simulink model "CLA_Sample"  (R2022b)
settings: Solver=FixedStepAuto  StartTime=0.0  StopTime=Inf  RelTol=1e-3  EnableMultiTasking=on
model workspace (MAT data in the model file):
  ADC_Gain = 1241.21212121
  DAC_Gain = 0.000805860805861
  Inductor_Current_Divider_Gain_Phase_A = 33.4
  Inductor_Current_Divider_Gain_Phase_B = 33.4
  Vbulk_Divider_Gain = 276.854928018
  Vin_Divider_Gain = 556.17352614
undefined symbols (not defined in the file or in its folder): GPTRIP1SEL, GPTRIP2SEL, SCI_A_Transmit, SCI_A_Transmit_Current_Suffix, SCI_A_Transmit_one_shot_Suffix, SCI_A_Transmit_Polarity_Suffix, SCI_A_Transmit_relay_Suffix, SCI_A_Transmit_Vbulk_Suffix, SCI_A_Transmit_Vin_rms_Suffix, SCI_A_Transmit_Vin_Suffix, SCI_A_Transmit_Vmid_Suffix, SCI_A_Transmit_Vp_Suffix, SCI_A_Transmit_Vpfc_Suffix, TZ1, TZ2
libraries: c280xlib x33, simulink x17, c2802xlib x15, c2000lib x1, c2806xlib x1
(part 4 of 5)

== system CLA_Sample/Calibration,RMS, Fault Protection @5kHz/Fault checking/If Action Subsystem/PFC_en_update_Phase_C ==
  function : TriggerPort  TriggerType=function-call  VariantControl=(inherit)
  Chart : Stateflow chart  TreatAsAtomicUnit=on
  Constant : Constant
  Data Store Read : DataStoreRead  Commented=on  DataStoreName=counter_Relay  IndexOptions=Index vector (dialog)  Indices=1  OutputSizes=1
  Data Store Read1 : DataStoreRead  DataStoreName=Vin_UVP_Flag_Phase_C  IndexOptions=Index vector (dialog)  Indices=1  OutputSizes=1
  Data Store Read2 : DataStoreRead  DataStoreName=Vin_OVP_Flag_Phase_C  IndexOptions=Index vector (dialog)  Indices=1  OutputSizes=1
  Data Store Read4 : DataStoreRead  DataStoreName=Iin_OCP_Flag_phase_C  IndexOptions=Index vector (dialog)  Indices=1  OutputSizes=1
  Data Store Write : DataStoreWrite  DataStoreName=PFC_en_Phase_C  IndexOptions=Index vector (dialog)  Indices=1  OutputSizes=1
  Data Store Write1 : DataStoreWrite  DataStoreName=PFC_en1  IndexOptions=Index vector (dialog)  Indices=1  OutputSizes=1
  Data Store Write2 : DataStoreWrite  Commented=on  DataStoreName=counter_Relay  IndexOptions=Index vector (dialog)  Indices=1  OutputSizes=1
  Product : Product  Commented=on
  wires:
  Chart/2(PFC_en1) -> Data Store Write1/1
  Data Store Read1/1 -> Chart/1(Vin_UVP_Flag)
  Data Store Read/1 -> Product/2
  Product/1 -> Data Store Write2/1
  Chart/1(PFC_en) -> Product/1, Data Store Write/1
  Data Store Read2/1 -> Chart/2(Vin_OVP_Flag)
  Data Store Read4/1 -> Chart/3(Iin_OCP_Flag)

== system CLA_Sample/Calibration,RMS, Fault Protection @5kHz/Fault checking/If Action Subsystem/Phase_A_Fault ==
  function : TriggerPort  TriggerType=function-call  VariantControl=(inherit)
  "Fault Check (Input OVP)_Phase_A " : Subsystem  TreatAsAtomicUnit=on
  "Fault Check (Input UVP)_Phase_A " : Subsystem  TreatAsAtomicUnit=on
  Function-Call Generator : simulink/Ports & Subsystems/Function-Call Generator  sample_time=-1  numberOfIterations=1  DisallowWideOutput=off
  Function-Call Split : FunctionCallSplit  IconShape=distinctive  NumOutputPorts=3  OutputPortLayout=default
  Input current_OCP_Phase_A : Subsystem  TreatAsAtomicUnit=on
  wires:
  Function-Call Generator/1 -> Function-Call Split/1
  Function-Call Split/1 -> "Fault Check (Input UVP)_Phase_A "/Trigger
  Function-Call Split/2 -> "Fault Check (Input OVP)_Phase_A "/Trigger
  Function-Call Split/3 -> Input current_OCP_Phase_A/Trigger

== system CLA_Sample/Calibration,RMS, Fault Protection @5kHz/Fault checking/If Action Subsystem/Phase_B_Fault ==
  function : TriggerPort  TriggerType=function-call  VariantControl=(inherit)
  Fault Check (Input OVP)_Phase_B : Subsystem  TreatAsAtomicUnit=on
  Fault Check (Input UVP)_Phase_B : Subsystem  TreatAsAtomicUnit=on
  Function-Call Generator : simulink/Ports & Subsystems/Function-Call Generator  sample_time=-1  numberOfIterations=1  DisallowWideOutput=off
  Function-Call Split : FunctionCallSplit  IconShape=distinctive  NumOutputPorts=3  OutputPortLayout=default
  Input current_OCP_Phase_B : Subsystem  TreatAsAtomicUnit=on
  wires:
  Function-Call Generator/1 -> Function-Call Split/1
  Function-Call Split/1 -> Fault Check (Input UVP)_Phase_B/Trigger
  Function-Call Split/2 -> Fault Check (Input OVP)_Phase_B/Trigger
  Function-Call Split/3 -> Input current_OCP_Phase_B/Trigger

== system CLA_Sample/Calibration,RMS, Fault Protection @5kHz/Fault checking/If Action Subsystem/Phase_C_Fault ==
  function : TriggerPort  TriggerType=function-call  VariantControl=(inherit)
  Fault Check (Input OVP)_Phase_C : Subsystem  TreatAsAtomicUnit=on
  Fault Check (Input UVP)_Phase_C : Subsystem  TreatAsAtomicUnit=on
  Function-Call Generator : simulink/Ports & Subsystems/Function-Call Generator  sample_time=-1  numberOfIterations=1  DisallowWideOutput=off
  Function-Call Split : FunctionCallSplit  IconShape=distinctive  NumOutputPorts=3  OutputPortLayout=default
  Input current_OCP_Phase_C : Subsystem  TreatAsAtomicUnit=on
  wires:
  Function-Call Generator/1 -> Function-Call Split/1
  Function-Call Split/1 -> Fault Check (Input UVP)_Phase_C/Trigger
  Function-Call Split/2 -> Fault Check (Input OVP)_Phase_C/Trigger
  Function-Call Split/3 -> Input current_OCP_Phase_C/Trigger

== system CLA_Sample/Calibration,RMS, Fault Protection @5kHz/Polarity & Near Zero check/Polarity_Near_zero_Phase_A/Volt to Number ==
  In1 : Inport
  Gain : Gain  Gain=ADC_Gain
  Gain1 : Gain  Gain=1/Vin_Divider_Gain
  Out1 : Outport
  wires:
  Gain1/1 -> Gain/1
  In1/1 -> Gain1/1
  Gain/1 -> Out1/1

== system CLA_Sample/Calibration,RMS, Fault Protection @5kHz/Polarity & Near Zero check/Polarity_Near_zero_Phase_B/Volt to Number ==
  In1 : Inport
  Gain : Gain  Gain=ADC_Gain
  Gain1 : Gain  Gain=1/Vin_Divider_Gain
  Out1 : Outport
  wires:
  Gain1/1 -> Gain/1
  In1/1 -> Gain1/1
  Gain/1 -> Out1/1

== system CLA_Sample/Calibration,RMS, Fault Protection @5kHz/Polarity & Near Zero check/Polarity_Near_zero_Phase_C/Volt to Number ==
  In1 : Inport
  Gain : Gain  Gain=ADC_Gain
  Gain1 : Gain  Gain=1/Vin_Divider_Gain
  Out1 : Outport
  wires:
  Gain1/1 -> Gain/1
  In1/1 -> Gain1/1
  Gain/1 -> Out1/1

== system CLA_Sample/Calibration,RMS, Fault Protection @5kHz/Relay control/Subsystem/ADC Gain2 ==
  In1 : Inport
  Gain : Gain  Gain=ADC_Gain
  Gain1 : Gain  Gain=1/Vin_Divider_Gain
  Out1 : Outport
  wires:
  Gain1/1 -> Gain/1
  In1/1 -> Gain1/1
  Gain/1 -> Out1/1

== system CLA_Sample/Calibration,RMS, Fault Protection @5kHz/Relay control/Subsystem/ADC Gain3 ==
  In1 : Inport
  Gain : Gain  Gain=ADC_Gain
  Gain1 : Gain  Gain=1/Vin_Divider_Gain
  Out1 : Outport
  wires:
  Gain1/1 -> Gain/1
  In1/1 -> Gain1/1
  Gain/1 -> Out1/1

== system CLA_Sample/Calibration,RMS, Fault Protection @5kHz/Voltage RMS//Averag Calculation/Phase_A/RMS Current Calculation_Phase_A ==
  note: RMS Voltage Calculation
  function : TriggerPort  TriggerType=function-call  VariantControl=(inherit)
  Chart : Stateflow chart  TreatAsAtomicUnit=on
  Data Store Read2 : DataStoreRead  DataStoreName=Inductor_Current_ADC_Phase_A  IndexOptions=Index vector (dialog)  Indices=1  OutputSizes=1
  Data Store Read5 : DataStoreRead  DataStoreName=Inductor_Current_1_65_ADC_Phase_A  IndexOptions=Index vector (dialog)  Indices=1  OutputSizes=1
  Data Store Write : DataStoreWrite  DataStoreName=Iin_rms_Phase_A  IndexOptions=Index vector (dialog)  Indices=1  OutputSizes=1
  Data Store Write1 : DataStoreWrite  DataStoreName=Iin_peak_Phase_A  IndexOptions=Index vector (dialog)  Indices=1  OutputSizes=1
  Gain1 : Gain  Gain=DAC_Gain
  Gain2 : Gain  Gain=DAC_Gain
  Gain3 : Gain  Gain=Inductor_Current_Divider_Gain_Phase_B
  Gain4 : Gain  Gain=Inductor_Current_Divider_Gain_Phase_B
  Gain5 : Gain  Gain=100
  Gain6 : Gain  Gain=100
  Subtract2 : Sum  Inputs=+-
  wires:
  Data Store Read2/1 -> Subtract2/1
  Data Store Read5/1 -> Subtract2/2
  Subtract2/1 -> Chart/1(input)
  Gain2/1 -> Gain3/1
  Chart/2(Vrms) -> Gain2/1
  Gain3/1 -> Gain6/1
  Gain6/1 -> Data Store Write/1
  Gain4/1 -> Gain5/1
  Gain1/1 -> Gain4/1
  Chart/1(Vpeak) -> Gain1/1
  Gain5/1 -> Data Store Write1/1

== system CLA_Sample/Calibration,RMS, Fault Protection @5kHz/Voltage RMS//Averag Calculation/Phase_A/RMS Voltage Calculation_Phase_A ==
  note: RMS Voltage Calculation
  function : TriggerPort  TriggerType=function-call  VariantControl=(inherit)
  Chart : Stateflow chart  TreatAsAtomicUnit=on
  Data Store Read2 : DataStoreRead  DataStoreName=Vin_ADC_Average_Phase_A  IndexOptions=Index vector (dialog)  Indices=1  OutputSizes=1
  Data Store Read5 : DataStoreRead  DataStoreName=Vin_1_65_ADC_Phase_A  IndexOptions=Index vector (dialog)  Indices=1  OutputSizes=1
  Data Store Write1 : DataStoreWrite  DataStoreName=Vin_peak_Phase_A  IndexOptions=Index vector (dialog)  Indices=1  OutputSizes=1
  Data Store Write2 : DataStoreWrite  DataStoreName=Vin_rms_Phase_A  IndexOptions=Index vector (dialog)  Indices=1  OutputSizes=1
  Data Store Write3 : DataStoreWrite  DataStoreName=Vin_peak_ADC_Phase_A  IndexOptions=Index vector (dialog)  Indices=1  OutputSizes=1
  Data Store Write4 : DataStoreWrite  DataStoreName=Vin_rms_ADC  IndexOptions=Index vector (dialog)  Indices=1  OutputSizes=1
  Digital Output : c280xlib/Digital Output  Commented=on  GPIO_Number=GPIO16~GPIO23  GPIO_Bit0=off  GPIO_BIT0_Toggle=off  GPIO_Bit1=off  GPIO_BIT1_Toggle=off  GPIO_Bit2=off  GPIO_BIT2_Toggle=off  GPIO_Bit3=off  GPIO_BIT3_Toggle=off  GPIO_Bit4=off  GPIO_BIT4_Toggle=off  GPIO_Bit5=off  GPIO_BIT5_Toggle=off  GPIO_Bit6=on  GPIO_BIT6_Toggle=off  GPIO_Bit7=off  GPIO_BIT7_Toggle=off
  Gain6 : Gain  Gain=DAC_Gain
  Gain7 : Gain  Gain=Vin_Divider_Gain  OutDataTypeStr=double
  Gain8 : Gain  Gain=DAC_Gain
  Gain9 : Gain  Gain=Vin_Divider_Gain  OutDataTypeStr=double
  Subtract2 : Sum  Inputs=+-
  wires:
  Chart/1(Vpeak) -> Data Store Write3/1, Gain8/1
  Chart/2(Vrms) -> Gain6/1, Data Store Write4/1
  Gain7/1 -> Data Store Write2/1
  Data Store Read2/1 -> Subtract2/1
  Gain8/1 -> Gain9/1
  Gain6/1 -> Gain7/1
  Data Store Read5/1 -> Subtract2/2
  Gain9/1 -> Data Store Write1/1
  Subtract2/1 -> Chart/1(input)

== system CLA_Sample/Calibration,RMS, Fault Protection @5kHz/Voltage RMS//Averag Calculation/Phase_A/Vin_ADC Averaging_Phase_A ==
  note: Low pass filter :
      | 1kHz bandwidth with 5kHz switching freq
  function : TriggerPort  TriggerType=function-call  VariantControl=(inherit)
  Chart1 : Stateflow chart  TreatAsAtomicUnit=on
  Constant1 : Constant  Value=0.38586954
  Constant2 : Constant  Value=0.38586954
  Constant3 : Constant  Value=-0.22826091
  Data Store Read3 : DataStoreRead  DataStoreName=Vin_ADC_Phase_A  IndexOptions=Index vector (dialog)  Indices=1  OutputSizes=1
  Vin_ADC_Average : DataStoreWrite  DataStoreName=Vin_ADC_Average_Phase_A  IndexOptions=Index vector (dialog)  Indices=1  OutputSizes=1
  wires:
  Constant3/1 -> [a1]
  Constant1/1 -> [b0]
  Constant2/1 -> [b1]
  [a1] -> Chart1/4(a1)
  [b1] -> Chart1/3(b1)
  [b0] -> Chart1/2(b0)
  Data Store Read3/1 -> Chart1/1(input_u)
  Chart1/1(output_y) -> Vin_ADC_Average/1

== system CLA_Sample/Calibration,RMS, Fault Protection @5kHz/Voltage RMS//Averag Calculation/Phase_B/RMS Current Calculation_Phase_B ==
  note: RMS Voltage Calculation
  function : TriggerPort  TriggerType=function-call  VariantControl=(inherit)
  Chart : Stateflow chart  TreatAsAtomicUnit=on
  Data Store Read2 : DataStoreRead  DataStoreName=Inductor_Current_ADC_Phase_B  IndexOptions=Index vector (dialog)  Indices=1  OutputSizes=1
  Data Store Read5 : DataStoreRead  DataStoreName=Inductor_Current_1_65_ADC_Phase_B  IndexOptions=Index vector (dialog)  Indices=1  OutputSizes=1
  Data Store Write : DataStoreWrite  DataStoreName=Iin_rms_Phase_B  IndexOptions=Index vector (dialog)  Indices=1  OutputSizes=1
  Data Store Write1 : DataStoreWrite  DataStoreName=Iin_peak_Phase_B  IndexOptions=Index vector (dialog)  Indices=1  OutputSizes=1
  Gain1 : Gain  Gain=DAC_Gain
  Gain2 : Gain  Gain=DAC_Gain
  Gain3 : Gain  Gain=Inductor_Current_Divider_Gain_Phase_B
  Gain4 : Gain  Gain=Inductor_Current_Divider_Gain_Phase_B
  Gain5 : Gain  Gain=100
  Gain6 : Gain  Gain=100
  Subtract2 : Sum  Inputs=+-
  wires:
  Data Store Read2/1 -> Subtract2/1
  Data Store Read5/1 -> Subtract2/2
  Subtract2/1 -> Chart/1(input)
  Gain2/1 -> Gain3/1
  Chart/2(Vrms) -> Gain2/1
  Gain3/1 -> Gain6/1
  Gain6/1 -> Data Store Write/1
  Gain5/1 -> Data Store Write1/1
  Gain1/1 -> Gain4/1
  Gain4/1 -> Gain5/1
  Chart/1(Vpeak) -> Gain1/1

== system CLA_Sample/Calibration,RMS, Fault Protection @5kHz/Voltage RMS//Averag Calculation/Phase_B/RMS Voltage Calculation_Phase_B ==
  note: RMS Voltage Calculation
  function : TriggerPort  TriggerType=function-call  VariantControl=(inherit)
  Chart : Stateflow chart  TreatAsAtomicUnit=on
  Data Store Read2 : DataStoreRead  DataStoreName=Vin_ADC_Average_Phase_B  IndexOptions=Index vector (dialog)  Indices=1  OutputSizes=1
  Data Store Read5 : DataStoreRead  DataStoreName=Vin_1_65_ADC_Phase_B  IndexOptions=Index vector (dialog)  Indices=1  OutputSizes=1
  Data Store Write1 : DataStoreWrite  DataStoreName=Vin_peak_Phase_B  IndexOptions=Index vector (dialog)  Indices=1  OutputSizes=1
  Data Store Write2 : DataStoreWrite  DataStoreName=Vin_rms_Phase_B  IndexOptions=Index vector (dialog)  Indices=1  OutputSizes=1
  Data Store Write3 : DataStoreWrite  DataStoreName=Vin_peak_ADC_Phase_B  IndexOptions=Index vector (dialog)  Indices=1  OutputSizes=1
  Data Store Write4 : DataStoreWrite  DataStoreName=Vin_rms_ADC  IndexOptions=Index vector (dialog)  Indices=1  OutputSizes=1
  Gain6 : Gain  Gain=DAC_Gain
  Gain7 : Gain  Gain=Vin_Divider_Gain  OutDataTypeStr=double
  Gain8 : Gain  Gain=DAC_Gain
  Gain9 : Gain  Gain=Vin_Divider_Gain  OutDataTypeStr=double
  Subtract2 : Sum  Inputs=+-
  wires:
  Chart/1(Vpeak) -> Data Store Write3/1, Gain8/1
  Chart/2(Vrms) -> Gain6/1, Data Store Write4/1
  Gain7/1 -> Data Store Write2/1
  Data Store Read2/1 -> Subtract2/1
  Gain8/1 -> Gain9/1
  Gain6/1 -> Gain7/1
  Data Store Read5/1 -> Subtract2/2
  Gain9/1 -> Data Store Write1/1
  Subtract2/1 -> Chart/1(input)

== system CLA_Sample/Calibration,RMS, Fault Protection @5kHz/Voltage RMS//Averag Calculation/Phase_B/Vin_ADC Averaging_Phase_B ==
  note: Low pass filter :
      | 1kHz bandwidth with 5kHz switching freq
  function : TriggerPort  TriggerType=function-call  VariantControl=(inherit)
  Chart1 : Stateflow chart  TreatAsAtomicUnit=on
  Constant1 : Constant  Value=0.38586954
  Constant2 : Constant  Value=0.38586954
  Constant3 : Constant  Value=-0.22826091
  Data Store Read3 : DataStoreRead  DataStoreName=Vin_ADC_Phase_B  IndexOptions=Index vector (dialog)  Indices=1  OutputSizes=1
  Vin_ADC_Average : DataStoreWrite  DataStoreName=Vin_ADC_Average_Phase_B  IndexOptions=Index vector (dialog)  Indices=1  OutputSizes=1
  wires:
  Constant3/1 -> [a1]
  Constant1/1 -> [b0]
  Constant2/1 -> [b1]
  [a1] -> Chart1/4(a1)
  [b1] -> Chart1/3(b1)
  [b0] -> Chart1/2(b0)
  Data Store Read3/1 -> Chart1/1(input_u)
  Chart1/1(output_y) -> Vin_ADC_Average/1

== system CLA_Sample/Calibration,RMS, Fault Protection @5kHz/Voltage RMS//Averag Calculation/Phase_C/RMS Current Calculation_Phase_C ==
  note: RMS Voltage Calculation
  function : TriggerPort  TriggerType=function-call  VariantControl=(inherit)
  Chart : Stateflow chart  TreatAsAtomicUnit=on
  Data Store Read2 : DataStoreRead  DataStoreName=Inductor_Current_ADC_Phase_C  IndexOptions=Index vector (dialog)  Indices=1  OutputSizes=1
  Data Store Read5 : DataStoreRead  DataStoreName=Inductor_Current_1_65_ADC_Phase_C  IndexOptions=Index vector (dialog)  Indices=1  OutputSizes=1
  Data Store Write : DataStoreWrite  DataStoreName=Iin_rms_Phase_C  IndexOptions=Index vector (dialog)  Indices=1  OutputSizes=1
  Data Store Write1 : DataStoreWrite  DataStoreName=Iin_peak_Phase_C  IndexOptions=Index vector (dialog)  Indices=1  OutputSizes=1
  Gain1 : Gain  Gain=DAC_Gain
  Gain2 : Gain  Gain=DAC_Gain
  Gain3 : Gain  Gain=Inductor_Current_Divider_Gain_Phase_B
  Gain4 : Gain  Gain=Inductor_Current_Divider_Gain_Phase_B
  Gain5 : Gain  Gain=100
  Gain6 : Gain  Gain=100
  Subtract2 : Sum  Inputs=+-
  wires:
  Data Store Read2/1 -> Subtract2/1
  Data Store Read5/1 -> Subtract2/2
  Subtract2/1 -> Chart/1(input)
  Gain2/1 -> Gain3/1
  Chart/2(Vrms) -> Gain2/1
  Gain3/1 -> Gain6/1
  Gain6/1 -> Data Store Write/1
  Gain5/1 -> Data Store Write1/1
  Gain1/1 -> Gain4/1
  Gain4/1 -> Gain5/1
  Chart/1(Vpeak) -> Gain1/1

== system CLA_Sample/Calibration,RMS, Fault Protection @5kHz/Voltage RMS//Averag Calculation/Phase_C/RMS Voltage Calculation_Phase_C ==
  note: RMS Voltage Calculation
  function : TriggerPort  TriggerType=function-call  VariantControl=(inherit)
  Chart : Stateflow chart  TreatAsAtomicUnit=on
  Data Store Read2 : DataStoreRead  DataStoreName=Vin_ADC_Average_Phase_C  IndexOptions=Index vector (dialog)  Indices=1  OutputSizes=1
  Data Store Read5 : DataStoreRead  DataStoreName=Vin_1_65_ADC_Phase_C  IndexOptions=Index vector (dialog)  Indices=1  OutputSizes=1
  Data Store Write1 : DataStoreWrite  DataStoreName=Vin_peak_Phase_C  IndexOptions=Index vector (dialog)  Indices=1  OutputSizes=1
  Data Store Write2 : DataStoreWrite  DataStoreName=Vin_rms_Phase_C  IndexOptions=Index vector (dialog)  Indices=1  OutputSizes=1
  Data Store Write3 : DataStoreWrite  DataStoreName=Vin_peak_ADC_Phase_C  IndexOptions=Index vector (dialog)  Indices=1  OutputSizes=1
  Data Store Write4 : DataStoreWrite  DataStoreName=Vin_rms_ADC  IndexOptions=Index vector (dialog)  Indices=1  OutputSizes=1
  Gain6 : Gain  Gain=DAC_Gain
  Gain7 : Gain  Gain=Vin_Divider_Gain  OutDataTypeStr=double
  Gain8 : Gain  Gain=DAC_Gain
  Gain9 : Gain  Gain=Vin_Divider_Gain  OutDataTypeStr=double
  Subtract2 : Sum  Inputs=+-
  wires:
  Chart/1(Vpeak) -> Data Store Write3/1, Gain8/1
  Chart/2(Vrms) -> Gain6/1, Data Store Write4/1
  Gain7/1 -> Data Store Write2/1
  Data Store Read2/1 -> Subtract2/1
  Gain8/1 -> Gain9/1
  Gain6/1 -> Gain7/1
  Data Store Read5/1 -> Subtract2/2
  Gain9/1 -> Data Store Write1/1
  Subtract2/1 -> Chart/1(input)

== system CLA_Sample/Calibration,RMS, Fault Protection @5kHz/Voltage RMS//Averag Calculation/Phase_C/Vin_ADC Averaging_Phase_C ==
  note: Low pass filter :
      | 1kHz bandwidth with 5kHz switching freq
  function : TriggerPort  TriggerType=function-call  VariantControl=(inherit)
  Chart1 : Stateflow chart  TreatAsAtomicUnit=on
  Constant1 : Constant  Value=0.38586954
  Constant2 : Constant  Value=0.38586954
  Constant3 : Constant  Value=-0.22826091
  Data Store Read3 : DataStoreRead  DataStoreName=Vin_ADC_Phase_C  IndexOptions=Index vector (dialog)  Indices=1  OutputSizes=1
  Vin_ADC_Average : DataStoreWrite  DataStoreName=Vin_ADC_Average_Phase_C  IndexOptions=Index vector (dialog)  Indices=1  OutputSizes=1
  wires:
  Constant3/1 -> [a1]
  Constant1/1 -> [b0]
  Constant2/1 -> [b1]
  [a1] -> Chart1/4(a1)
  [b1] -> Chart1/3(b1)
  [b0] -> Chart1/2(b0)
  Data Store Read3/1 -> Chart1/1(input_u)
  Chart1/1(output_y) -> Vin_ADC_Average/1

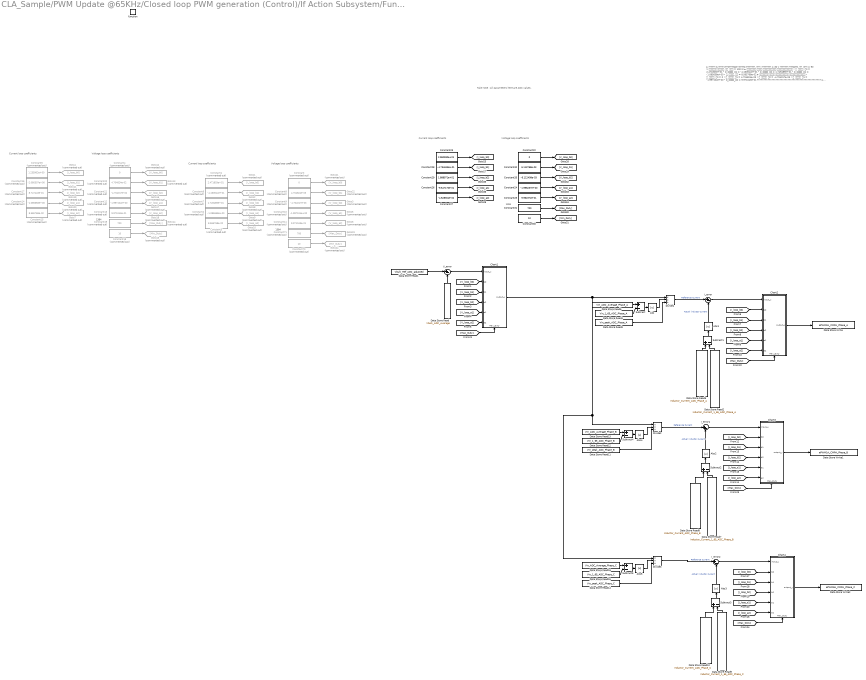
== system CLA_Sample/PWM Update @65KHz/Closed loop PWM generation (Control)/If Action Subsystem/Function-Call Subsystem ==
  note: 1384
  note: Voltage loop coefficients
  note: 1384
  note: Current loop coefficients
  note: Voltage loop coefficients
  note: Voltage loop coefficients
  note: ► 𝑷𝒍𝒂𝒏𝒕 & 𝑳𝒐𝒂𝒅 𝒑𝒂𝒓𝒂𝒎𝒆𝒕𝒆𝒓𝒔
      | 𝑰𝒏𝒑𝒖𝒕 𝒗𝒐𝒍𝒕𝒂𝒈𝒆, 𝑽𝒊𝒏_𝒏𝒐𝒎𝒊𝒏𝒂𝒍 = 30 V
      | 𝑶𝒖𝒕𝒑𝒖𝒕 𝒗𝒐𝒍𝒕𝒂𝒈𝒆, 𝑽𝒐_𝑷𝑭𝑪 = 90 V
      | 𝑶𝒖𝒕𝒑𝒖𝒕 𝒑𝒐𝒘𝒆𝒓, 𝑷𝒐_𝑷𝑭𝑪 = 100 W
      |
      | ► 𝑪𝒖𝒓𝒓𝒆𝒏𝒕 𝒍𝒐𝒐𝒑 𝒄𝒐𝒏𝒕𝒓𝒐𝒍𝒍𝒆𝒓 𝒄𝒐𝒆𝒇𝒇𝒊𝒄𝒊𝒆𝒏𝒕𝒔
      | • 𝑰_𝒍𝒐𝒐𝒑_𝒃0 = 2.471803e+01
      | • 𝑰_𝒍𝒐𝒐𝒑_𝒃1 = -4.160614e+01
      | • 𝑰_𝒍𝒐𝒐𝒑_𝒃2 = 1.749489e+01
      | • 𝑰_𝒍𝒐𝒐𝒑_𝒂1 = -1.085658e+00
      | • 𝑰_𝒍𝒐𝒐𝒑_𝒂2 = 8.565768e-02
      |
      | ► 𝑽𝒐𝒍𝒕𝒂𝒈𝒆 𝒍𝒐𝒐𝒑 𝒄𝒐𝒏𝒕𝒓𝒐𝒍𝒍𝒆𝒓 𝒄𝒐𝒆𝒇𝒇𝒊𝒄𝒊𝒆𝒏𝒕𝒔
      | • 𝑽_𝒍𝒐𝒐𝒑_𝒃0 = 0
      | • 𝑽_𝒍𝒐𝒐𝒑_𝒃1 = 4.704824e-03
      | • 𝑽_𝒍𝒐𝒐𝒑_𝒃2 = -4.704017e-03
      | • 𝑽_𝒍𝒐𝒐𝒑_𝒂1 = -1.997104e+00
      | • 𝑽_𝒍𝒐𝒐𝒑_𝒂2 = 9.971043e-01
      |
      | ************************************************
      | ► 𝑻𝒉𝒆 𝒇𝒐𝒓𝒎𝒂𝒕 𝒇𝒐𝒓 𝒄𝒐𝒆𝒇𝒇𝒊𝒄𝒊𝒆𝒏𝒕𝒔 𝒊𝒔 𝒔𝒉𝒐𝒘𝒏 𝒃𝒆𝒍𝒐𝒘.
      |
      | 𝒚(𝒌) = 𝒃0 𝒆(𝒌) + 𝒃1 𝒆(𝒌−1) + 𝒃2 𝒆(𝒌−2) − 𝒂1 𝒚(𝒌−1) − 𝒂2 𝒚(𝒌−2)
      |
      | ************************************************
      | ◘◘◘◘◘◘◘◘◘◘◘◘◘◘◘◘◘◘◘◘◘◘◘◘◘◘◘◘◘◘◘◘◘◘◘◘◘◘◘◘◘◘◘◘◘◘◘◘
  note: 1384
  note: Current loop coefficients
  note: Take note : All parameters here are ADC values.
  note: Current loop coefficients
  function : TriggerPort  TriggerType=function-call  VariantControl=(inherit)
  Abs{,1..5} (6 alike) : Abs  SaturateOnIntegerOverflow=off
  Chart1 : Stateflow chart  TreatAsAtomicUnit=on
      settings: PortSchema="{\"entries\":[{\"content\":{\"sides\":[{\"content\":{\"connectorIds\":[\"In2\",\"In3\",\"In4\",\"In5\",\"In6\",\"In7\"]},\"type\":\"ConnectorPlacement.EquallySpacedRectSide\",\"uuid\":\"98054acb-dc05-45b7-9e49-d1f1309a60af\"},{\"content\":{\"connectorIds\":[\"Out1\"],\"side\":\"RIGHT\"},\"type\":\"ConnectorPlacement.EquallySpacedRectSide\",\"uuid\":\"519c6a11-fba4-4420-9bc2-f24cec898983\"},{\"content\":{\"connectorIds\":[],\"side\":\"TOP\"},\"type\":\"ConnectorPlacement.EquallySpacedRectSide\",\"uuid\":\"37e92206-8070-4c6c-85b3-8eb12c5538cd\"},{\"content\":{\"connectorIds\":[\"In1\"],\"side\":\"BOTTOM\"},\"type\":\"ConnectorPlacement.EquallySpacedRectSide\",\"uuid\":\"a24e42b6-e88f-4c7d-a70a-f75d0d02a985\"}]},\"type\":\"ConnectorPlacement.EquallySpacedConnector\",\"uuid\":\"7d467722-ac20-43d4-98e5-7341f60d2894\"}],\"packageUris\":[\"http://schema.mathworks.com/mf0/Connector/R2020b\"],\"version\":\"1.0\"}"
  Chart2 : Stateflow chart  TreatAsAtomicUnit=on
      settings: PortSchema="{\"entries\":[{\"content\":{\"sides\":[{\"content\":{\"connectorIds\":[\"In2\",\"In3\",\"In4\",\"In5\",\"In6\",\"In7\"]},\"type\":\"ConnectorPlacement.EquallySpacedRectSide\",\"uuid\":\"98054acb-dc05-45b7-9e49-d1f1309a60af\"},{\"content\":{\"connectorIds\":[\"Out1\"],\"side\":\"RIGHT\"},\"type\":\"ConnectorPlacement.EquallySpacedRectSide\",\"uuid\":\"519c6a11-fba4-4420-9bc2-f24cec898983\"},{\"content\":{\"connectorIds\":[],\"side\":\"TOP\"},\"type\":\"ConnectorPlacement.EquallySpacedRectSide\",\"uuid\":\"37e92206-8070-4c6c-85b3-8eb12c5538cd\"},{\"content\":{\"connectorIds\":[\"In1\"],\"side\":\"BOTTOM\"},\"type\":\"ConnectorPlacement.EquallySpacedRectSide\",\"uuid\":\"c357f4bc-ad64-4f69-8a5c-2d122a217843\"}]},\"type\":\"ConnectorPlacement.EquallySpacedConnector\",\"uuid\":\"7d467722-ac20-43d4-98e5-7341f60d2894\"}],\"packageUris\":[\"http://schema.mathworks.com/mf0/Connector/R2020b\"],\"version\":\"1.0\"}"
  Chart3 : Stateflow chart  TreatAsAtomicUnit=on
      settings: PortSchema="{\"entries\":[{\"content\":{\"sides\":[{\"content\":{\"connectorIds\":[\"In2\",\"In3\",\"In4\",\"In5\",\"In6\",\"In7\"]},\"type\":\"ConnectorPlacement.EquallySpacedRectSide\",\"uuid\":\"98054acb-dc05-45b7-9e49-d1f1309a60af\"},{\"content\":{\"connectorIds\":[\"Out1\"],\"side\":\"RIGHT\"},\"type\":\"ConnectorPlacement.EquallySpacedRectSide\",\"uuid\":\"519c6a11-fba4-4420-9bc2-f24cec898983\"},{\"content\":{\"connectorIds\":[],\"side\":\"TOP\"},\"type\":\"ConnectorPlacement.EquallySpacedRectSide\",\"uuid\":\"37e92206-8070-4c6c-85b3-8eb12c5538cd\"},{\"content\":{\"connectorIds\":[\"In1\"],\"side\":\"BOTTOM\"},\"type\":\"ConnectorPlacement.EquallySpacedRectSide\",\"uuid\":\"2f414d73-99cb-441b-a85c-e16df8718e53\"}]},\"type\":\"ConnectorPlacement.EquallySpacedConnector\",\"uuid\":\"7d467722-ac20-43d4-98e5-7341f60d2894\"}],\"packageUris\":[\"http://schema.mathworks.com/mf0/Connector/R2020b\"],\"version\":\"1.0\"}"
  Chart4 : Stateflow chart  TreatAsAtomicUnit=on
      settings: PortSchema="{\"entries\":[{\"content\":{\"sides\":[{\"content\":{\"connectorIds\":[\"In2\",\"In3\",\"In4\",\"In5\",\"In6\",\"In7\"]},\"type\":\"ConnectorPlacement.EquallySpacedRectSide\",\"uuid\":\"98054acb-dc05-45b7-9e49-d1f1309a60af\"},{\"content\":{\"connectorIds\":[\"Out1\"],\"side\":\"RIGHT\"},\"type\":\"ConnectorPlacement.EquallySpacedRectSide\",\"uuid\":\"519c6a11-fba4-4420-9bc2-f24cec898983\"},{\"content\":{\"connectorIds\":[],\"side\":\"TOP\"},\"type\":\"ConnectorPlacement.EquallySpacedRectSide\",\"uuid\":\"37e92206-8070-4c6c-85b3-8eb12c5538cd\"},{\"content\":{\"connectorIds\":[\"In1\"],\"side\":\"BOTTOM\"},\"type\":\"ConnectorPlacement.EquallySpacedRectSide\",\"uuid\":\"3fbeedd5-4cc1-4149-822b-0a6b54a0fe71\"}]},\"type\":\"ConnectorPlacement.EquallySpacedConnector\",\"uuid\":\"7d467722-ac20-43d4-98e5-7341f60d2894\"}],\"packageUris\":[\"http://schema.mathworks.com/mf0/Connector/R2020b\"],\"version\":\"1.0\"}"
  Constant : Constant  Commented=on  Value=0
  Constant1 : Constant  Commented=on  Value=2.471803e+01
  Constant10 : Constant  Commented=on  Value=-1.997104e+00
  Constant11 : Constant  Commented=on  Value=9.971043e-01
  Constant12 : Constant  Commented=on  Value=-1.997104e+00
  Constant13 : Constant  Commented=on  Value=9.971043e-01
  Constant14 : Constant  Commented=on  Value=-1.085658e+00
  Constant15 : Constant  Commented=on  Value=8.565768e-02
  Constant16 : Constant  Commented=on  Value=-2.080307e+00
  Constant17 : Constant  Commented=on  Value=8.747443e-01
  Constant18 : Constant  Commented=on  Value=10  OutDataTypeStr=double
  Constant19 : Constant  Commented=on  Value=700  OutDataTypeStr=double
  Constant2 : Constant  Commented=on  Value=-1.085658e+00
  Constant20 : Constant  Commented=on  Value=4.704824e-02
  Constant21 : Constant  Commented=on  Value=-4.704017e-02
  Constant22 : Constant  Value=0
  Constant23 : Constant  Value=2.962930e+01
  Constant24 : Constant  Value=-1.996237e+00
  Constant25 : Constant  Value=9.962372e-01
  Constant26 : Constant  Value=-9.547170e-01
  Constant27 : Constant  Value=-4.528304e-02
  Constant28 : Constant  Value=-4.734618e+01
  Constant29 : Constant  Value=1.888971e+01
  Constant3 : Constant  Commented=on  Value=8.565768e-02
  Constant30 : Constant  Value=10  OutDataTypeStr=double
  Constant31 : Constant  Value=700  OutDataTypeStr=double
  Constant32 : Constant  Value=6.113768e-03
  Constant33 : Constant  Value=-6.112408e-03
  Constant4 : Constant  Commented=on  Value=0
  Constant5 : Constant  Commented=on  Value=1.235902e+00
  Constant6 : Constant  Commented=on  Value=-4.160614e+01
  Constant7 : Constant  Commented=on  Value=1.749489e+01
  Constant70 : Constant  Commented=on  Value=10  OutDataTypeStr=double
  Constant71 : Constant  Commented=on  Value=700  OutDataTypeStr=double
  Constant8 : Constant  Commented=on  Value=4.704824e-03
  Constant9 : Constant  Commented=on  Value=-4.704017e-03
  Data Store Read : DataStoreRead  DataStoreName=Vbulk_ADC_Average  IndexOptions=Index vector (dialog)  Indices=1  OutputSizes=1
  Data Store Read1 : DataStoreRead  DataStoreName=Vbulk_Ref_ADC_adjusted  IndexOptions=Index vector (dialog)  Indices=1  OutputSizes=1
  Data Store Read10 : DataStoreRead  DataStoreName=Inductor_Current_ADC_Phase_C  IndexOptions=Index vector (dialog)  Indices=1  OutputSizes=1
  Data Store Read11 : DataStoreRead  DataStoreName=Vin_peak_ADC_Phase_B  IndexOptions=Index vector (dialog)  Indices=1  OutputSizes=1
  Data Store Read12 : DataStoreRead  DataStoreName=Vin_1_65_ADC_Phase_B  IndexOptions=Index vector (dialog)  Indices=1  OutputSizes=1
  Data Store Read13 : DataStoreRead  DataStoreName=Vin_ADC_Average_Phase_B  IndexOptions=Index vector (dialog)  Indices=1  OutputSizes=1
  Data Store Read14 : DataStoreRead  DataStoreName=Vin_peak_ADC_Phase_C  IndexOptions=Index vector (dialog)  Indices=1  OutputSizes=1
  Data Store Read15 : DataStoreRead  DataStoreName=Vin_1_65_ADC_Phase_C  IndexOptions=Index vector (dialog)  Indices=1  OutputSizes=1
  Data Store Read16 : DataStoreRead  DataStoreName=Vin_ADC_Average_Phase_C  IndexOptions=Index vector (dialog)  Indices=1  OutputSizes=1
  Data Store Read2 : DataStoreRead  DataStoreName=Inductor_Current_1_65_ADC_Phase_A  IndexOptions=Index vector (dialog)  Indices=1  OutputSizes=1
  Data Store Read3 : DataStoreRead  DataStoreName=Vin_peak_ADC_Phase_A  IndexOptions=Index vector (dialog)  Indices=1  OutputSizes=1
  Data Store Read4 : DataStoreRead  DataStoreName=Vin_1_65_ADC_Phase_A  IndexOptions=Index vector (dialog)  Indices=1  OutputSizes=1
  Data Store Read5 : DataStoreRead  DataStoreName=Inductor_Current_ADC_Phase_A  IndexOptions=Index vector (dialog)  Indices=1  OutputSizes=1
  Data Store Read6 : DataStoreRead  DataStoreName=Vin_ADC_Average_Phase_A  IndexOptions=Index vector (dialog)  Indices=1  OutputSizes=1
  Data Store Read7 : DataStoreRead  DataStoreName=Inductor_Current_1_65_ADC_Phase_B  IndexOptions=Index vector (dialog)  Indices=1  OutputSizes=1
  Data Store Read8 : DataStoreRead  DataStoreName=Inductor_Current_ADC_Phase_B  IndexOptions=Index vector (dialog)  Indices=1  OutputSizes=1
  Data Store Read9 : DataStoreRead  DataStoreName=Inductor_Current_1_65_ADC_Phase_C  IndexOptions=Index vector (dialog)  Indices=1  OutputSizes=1
  Data Store Write : DataStoreWrite  DataStoreName=ePWM2A_CMPA_Phase_A  IndexOptions=Index vector (dialog)  Indices=1  OutputSizes=1
  Data Store Write1 : DataStoreWrite  DataStoreName=ePWM1A_CMPA_Phase_B  IndexOptions=Index vector (dialog)  Indices=1  OutputSizes=1
  Data Store Write2 : DataStoreWrite  DataStoreName=ePWM3A_CMPA_Phase_C  IndexOptions=Index vector (dialog)  Indices=1  OutputSizes=1
  Divide1 : Product  Inputs=**/  RndMeth=Zero  SaturateOnIntegerOverflow=on
  Divide2 : Product  Inputs=**/  RndMeth=Zero  SaturateOnIntegerOverflow=on
  Divide3 : Product  Inputs=**/  RndMeth=Zero  SaturateOnIntegerOverflow=on
  Goto1 : Goto  Commented=on  GotoTag=I_loop_b0
  Goto10 : Goto  Commented=on  GotoTag=I_loop_a2
  Goto11 : Goto  Commented=on  GotoTag=I_loop_b1
  Goto12 : Goto  Commented=on  GotoTag=V_loop_b0
  Goto13 : Goto  Commented=on  GotoTag=V_loop_b1
  Goto14 : Goto  Commented=on  GotoTag=Max_Duty
  Goto15 : Goto  Commented=on  GotoTag=Min_Duty
  Goto16 : Goto  Commented=on  GotoTag=V_loop_b2
  Goto17 : Goto  Commented=on  GotoTag=V_loop_a1
  Goto18 : Goto  Commented=on  GotoTag=V_loop_a2
  Goto19 : Goto  Commented=on  GotoTag=I_loop_b2
  Goto2 : Goto  Commented=on  GotoTag=I_loop_b1
  Goto20 : Goto  Commented=on  GotoTag=I_loop_a1
  Goto21 : Goto  Commented=on  GotoTag=V_loop_b0
  Goto22 : Goto  Commented=on  GotoTag=V_loop_b1
  Goto23 : Goto  Commented=on  GotoTag=Max_Duty
  Goto24 : Goto  Commented=on  GotoTag=Min_Duty
  Goto3 : Goto  Commented=on  GotoTag=V_loop_b2
  Goto4 : Goto  Commented=on  GotoTag=I_loop_b0
  Goto5 : Goto  Commented=on  GotoTag=V_loop_a1
  Goto6 : Goto  Commented=on  GotoTag=V_loop_a2
  Goto7 : Goto  Commented=on  GotoTag=I_loop_a2
  Goto8 : Goto  Commented=on  GotoTag=I_loop_b2
  Goto9 : Goto  Commented=on  GotoTag=I_loop_a1
  I_error : Sum  Inputs=|+-  AccumDataTypeStr=double  OutDataTypeStr=double
  I_error1 : Sum  Inputs=|+-  AccumDataTypeStr=double  OutDataTypeStr=double
  I_error2 : Sum  Inputs=|+-  AccumDataTypeStr=double  OutDataTypeStr=double
  Subtract{,1..5} (6 alike) : Sum  Inputs=+-
  V_error : Sum  Inputs=|+-  AccumDataTypeStr=double  OutDataTypeStr=double
  wires:
  Divide1/1 -> I_error/1  "Reference Current"
  [I_loop_a1] -> Chart4/6(a1)
  Chart1/1(output_y) -> Divide3/1, Divide2/1, Divide1/1
  Data Store Read5/1 -> Subtract1/1
  Constant22/1 -> [V_loop_b0]
  Constant32/1 -> [V_loop_b1]
  I_error2/1 -> Chart4/2(input_u)
  Subtract4/1 -> Abs4/1
  Constant14/1 -> Goto20/1
  Data Store Read11/1 -> Divide2/3
  Subtract5/1 -> Abs5/1
  Abs2/1 -> I_error1/2  "Actual inductor current"
  Constant25/1 -> [V_loop_a2]
  Data Store Read14/1 -> Divide3/3
  Data Store Read15/1 -> Subtract5/2
  Abs5/1 -> Divide3/2
  Divide3/1 -> I_error2/1  "Reference Current"
  [I_loop_b0] -> Chart3/3(b0)
  Constant33/1 -> [V_loop_b2]
  Constant71/1 -> Goto23/1
  [I_loop_b0] -> Chart2/3(b0)
  [V_loop_a1] -> Chart1/6(a1)
  Constant6/1 -> Goto2/1
  Subtract1/1 -> Abs1/1
  [V_loop_b2] -> Chart1/5(b2)
  Abs4/1 -> Divide2/2
  Constant/1 -> Goto21/1
  Chart4/1(output_y) -> Data Store Write2/1
  Data Store Read7/1 -> Subtract2/2
  Data Store Read8/1 -> Subtract2/1
  [I_loop_a2] -> Chart3/7(a2)
  Chart2/1(output_y) -> Data Store Write/1
  [I_loop_b2] -> Chart3/5(b2)
  [I_loop_b1] -> Chart3/4(b1)
  Data Store Read1/1 -> V_error/1
  [I_loop_a2] -> Chart2/7(a2)
  Subtract2/1 -> Abs2/1
  Constant10/1 -> Goto5/1
  Abs1/1 -> I_error/2  "Actual inductor current"
  Data Store Read2/1 -> Subtract1/2
  Subtract/1 -> Abs/1
  Constant2/1 -> Goto9/1
  Constant3/1 -> Goto10/1
  Constant9/1 -> Goto3/1
  Constant11/1 -> Goto6/1
  Constant8/1 -> Goto22/1
  Data Store Read4/1 -> Subtract/2
  Constant7/1 -> Goto8/1
  [I_loop_b1] -> Chart2/4(b1)
  Chart3/1(output_y) -> Data Store Write1/1
  [V_loop_b0] -> Chart1/3(b0)
  [Max_Duty] -> Chart3/1(Max_Duty)
  Data Store Read3/1 -> Divide1/3
  Constant70/1 -> Goto24/1
  Constant20/1 -> Goto13/1
  Data Store Read9/1 -> Subtract3/2
  Data Store Read10/1 -> Subtract3/1
  [I_loop_b0] -> Chart4/3(b0)
  [V_loop_a2] -> Chart1/7(a2)
  Constant13/1 -> Goto18/1
  [V_loop_b1] -> Chart1/4(b1)
  V_error/1 -> Chart1/2(input_u)
  [I_loop_a2] -> Chart4/7(a2)
  Constant16/1 -> Goto11/1
  [I_loop_a1] -> Chart2/6(a1)
  Constant21/1 -> Goto16/1
  [I_loop_a1] -> Chart3/6(a1)
  Constant15/1 -> Goto7/1
  Abs3/1 -> I_error2/2  "Actual inductor current"
  Constant12/1 -> Goto17/1
  Divide2/1 -> I_error1/1  "Reference Current"
  I_error/1 -> Chart2/2(input_u)
  Constant27/1 -> [I_loop_a2]
  Constant31/1 -> [Max_Duty]
  Subtract3/1 -> Abs3/1
  [Max_Duty] -> Chart1/1(Max_Duty)
  Constant5/1 -> Goto4/1
  I_error1/1 -> Chart3/2(input_u)
  [I_loop_b1] -> Chart4/4(b1)
  Constant18/1 -> Goto15/1
  [Max_Duty] -> Chart4/1(Max_Duty)
  Constant28/1 -> [I_loop_b1]
  [I_loop_b2] -> Chart2/5(b2)
  [Max_Duty] -> Chart2/1(Max_Duty)
  Constant26/1 -> [I_loop_a1]
  Data Store Read6/1 -> Subtract/1
  Constant30/1 -> [Min_Duty]
  Constant29/1 -> [I_loop_b2]
  Data Store Read13/1 -> Subtract4/1
  Constant19/1 -> Goto14/1
  Data Store Read/1 -> V_error/2
  Abs/1 -> Divide1/2
  Constant24/1 -> [V_loop_a1]
  Constant23/1 -> [I_loop_b0]
  Data Store Read16/1 -> Subtract5/1
  [I_loop_b2] -> Chart4/5(b2)
  Constant1/1 -> Goto1/1
  Data Store Read12/1 -> Subtract4/2
  Constant4/1 -> Goto12/1
  Constant17/1 -> Goto19/1

== system CLA_Sample/PWM Update @65KHz/Fixed Duty update_Phase_A/Archive/If Action Subsystem ==
  Action Port : ActionPort  ActionPortLabel=if(u1 ==0)
  Constant : Constant  Value=0
  Data Store Write : DataStoreWrite  DataStoreName=PWM_DutyNearzero  IndexOptions=Index vector (dialog)  Indices=1  OutputSizes=1
  wires:
  Constant/1 -> Data Store Write/1

== system CLA_Sample/PWM Update @65KHz/Fixed Duty update_Phase_A/Archive/If Action Subsystem1 ==
  In1 : Inport  OutDataTypeStr=double
  Action Port : ActionPort  ActionPortLabel=if(u1 ==1)
  Out1 : Outport  OutDataTypeStr=double
  wires:
  In1/1 -> Out1/1

== system CLA_Sample/PWM Update @65KHz/Fixed Duty update_Phase_A/Archive/If Action Subsystem2 ==
  In1 : Inport
  Action Port : ActionPort  ActionPortLabel=else
  Out1 : Outport
  wires:
  In1/1 -> Out1/1

== system CLA_Sample/PWM Update @65KHz/Fixed Duty update_Phase_A/Archive/If Action Subsystem3 ==
  Action Port : ActionPort  ActionPortLabel=else
  Data Store Read7 : DataStoreRead  DataStoreName=Polarity_Phase_A  IndexOptions=Index vector (dialog)  Indices=1  OutputSizes=1
  If Action Subsystem4 : Subsystem  TreatAsAtomicUnit=on
  If Action Subsystem5 : Subsystem  TreatAsAtomicUnit=on
  If2 : If  IfExpression=u1 ==1
  wires:
  Data Store Read7/1 -> If2/1
  If2/2 -> If Action Subsystem5/Action
  If2/1 -> If Action Subsystem4/Action

== system CLA_Sample/PWM Update @65KHz/Fixed Duty update_Phase_B/Archive/If Action Subsystem ==
  Action Port : ActionPort
  Constant : Constant  Value=0
  Data Store Write : DataStoreWrite  DataStoreName=PWM_DutyNearzero  IndexOptions=Index vector (dialog)  Indices=1  OutputSizes=1
  wires:
  Constant/1 -> Data Store Write/1

== system CLA_Sample/PWM Update @65KHz/Fixed Duty update_Phase_B/Archive/If Action Subsystem1 ==
  In1 : Inport  OutDataTypeStr=double
  Action Port : ActionPort
  Out1 : Outport  OutDataTypeStr=double
  wires:
  In1/1 -> Out1/1

== system CLA_Sample/PWM Update @65KHz/Fixed Duty update_Phase_B/Archive/If Action Subsystem2 ==
  In1 : Inport
  Action Port : ActionPort
  Out1 : Outport
  wires:
  In1/1 -> Out1/1

== system CLA_Sample/PWM Update @65KHz/Fixed Duty update_Phase_B/Archive/If Action Subsystem3 ==
  Action Port : ActionPort
  Data Store Read7 : DataStoreRead  DataStoreName=Polarity_Phase_A  IndexOptions=Index vector (dialog)  Indices=1  OutputSizes=1
  If Action Subsystem4 : Subsystem  TreatAsAtomicUnit=on
  If Action Subsystem5 : Subsystem  TreatAsAtomicUnit=on
  If2 : If  IfExpression=u1 ==1
  wires:
  Data Store Read7/1 -> If2/1
  If2/2 -> If Action Subsystem5/Action
  If2/1 -> If Action Subsystem4/Action

== system CLA_Sample/PWM Update @65KHz/Fixed Duty update_Phase_C/Archive/If Action Subsystem ==
  Action Port : ActionPort
  Constant : Constant  Value=0
  Data Store Write : DataStoreWrite  DataStoreName=PWM_DutyNearzero  IndexOptions=Index vector (dialog)  Indices=1  OutputSizes=1
  wires:
  Constant/1 -> Data Store Write/1

== system CLA_Sample/PWM Update @65KHz/Fixed Duty update_Phase_C/Archive/If Action Subsystem1 ==
  In1 : Inport  OutDataTypeStr=double
  Action Port : ActionPort
  Out1 : Outport  OutDataTypeStr=double
  wires:
  In1/1 -> Out1/1

== system CLA_Sample/PWM Update @65KHz/Fixed Duty update_Phase_C/Archive/If Action Subsystem2 ==
  In1 : Inport
  Action Port : ActionPort
  Out1 : Outport
  wires:
  In1/1 -> Out1/1

== system CLA_Sample/PWM Update @65KHz/Fixed Duty update_Phase_C/Archive/If Action Subsystem3 ==
  Action Port : ActionPort
  Data Store Read7 : DataStoreRead  DataStoreName=Polarity_Phase_A  IndexOptions=Index vector (dialog)  Indices=1  OutputSizes=1
  If Action Subsystem4 : Subsystem  TreatAsAtomicUnit=on
  If Action Subsystem5 : Subsystem  TreatAsAtomicUnit=on
  If2 : If  IfExpression=u1 ==1
  wires:
  Data Store Read7/1 -> If2/1
  If2/2 -> If Action Subsystem5/Action
  If2/1 -> If Action Subsystem4/Action

== system CLA_Sample/Calibration,RMS, Fault Protection @5kHz/Fault checking/If Action Subsystem/Phase_A_Fault/Fault Check (Input OVP)_Phase_A  ==
  note: "Von_Threshold" is set inside this state machine
  note: Fault Check (Input UVP)
  function : TriggerPort  TriggerType=function-call  VariantControl=(inherit)
  Chart1 : Stateflow chart  TreatAsAtomicUnit=on
  Data Store Read3 : DataStoreRead  DataStoreName=Vin_rms_Phase_A  IndexOptions=Index vector (dialog)  Indices=1  OutputSizes=1
  Data Store Write : DataStoreWrite  DataStoreName=Vin_OVP_Flag_Phase_A  IndexOptions=Index vector (dialog)  Indices=1  OutputSizes=1
  wires:
  Data Store Read3/1 -> Chart1/1(input)
  Chart1/1(Input_OVP_Flag) -> Data Store Write/1

== system CLA_Sample/Calibration,RMS, Fault Protection @5kHz/Fault checking/If Action Subsystem/Phase_A_Fault/Fault Check (Input UVP)_Phase_A  ==
  note: "Von_Threshold" is set inside this state machine
  note: Fault Check (Input UVP)
  function : TriggerPort  TriggerType=function-call  VariantControl=(inherit)
  Chart1 : Stateflow chart  TreatAsAtomicUnit=on
  Data Store Read3 : DataStoreRead  DataStoreName=Vin_rms_Phase_A  IndexOptions=Index vector (dialog)  Indices=1  OutputSizes=1
  Data Store Write : DataStoreWrite  DataStoreName=Vin_UVP_Flag_Phase_A  IndexOptions=Index vector (dialog)  Indices=1  OutputSizes=1
  wires:
  Data Store Read3/1 -> Chart1/1(input)
  Chart1/1(Input_UVP_Flag) -> Data Store Write/1

== system CLA_Sample/Calibration,RMS, Fault Protection @5kHz/Fault checking/If Action Subsystem/Phase_A_Fault/Input current_OCP_Phase_A ==
  note: Vbulk_OVP_Threshold initialized in Data Store Memory
  note: Output Voltage_Latch_OVP
  function : TriggerPort  TriggerType=function-call  VariantControl=(inherit)
  Abs : Abs  SaturateOnIntegerOverflow=off
  Chart2 : Stateflow chart  TreatAsAtomicUnit=on
  Data Store Read : DataStoreRead  DataStoreName=Inductor_Current_ADC_Phase_A  IndexOptions=Index vector (dialog)  Indices=1  OutputSizes=1
  Data Store Read1 : DataStoreRead  DataStoreName=Iin_OCP_Threshold  IndexOptions=Index vector (dialog)  Indices=1  OutputSizes=1
  Data Store Read3 : DataStoreRead  DataStoreName=Inductor_Current_1_65_ADC_Phase_A  IndexOptions=Index vector (dialog)  Indices=1  OutputSizes=1
  Data Store Write1 : DataStoreWrite  DataStoreName=Iin_OCP_Flag_phase_A  IndexOptions=Index vector (dialog)  Indices=1  OutputSizes=1
  Gain2 : Gain  Gain=0.00080586
  Gain3 : Gain  Gain=33.445
  Subtract2 : Sum  Inputs=+-
  wires:
  Gain3/1 -> Abs/1
  Data Store Read3/1 -> Subtract2/2
  Data Store Read/1 -> Subtract2/1
  Chart2/1(Iin_OCP_Flag) -> Data Store Write1/1
  Gain2/1 -> Gain3/1
  Subtract2/1 -> Gain2/1
  Abs/1 -> Chart2/1(input_Iin)
  Data Store Read1/1 -> Chart2/2("OCP_Threshold ")

== system CLA_Sample/Calibration,RMS, Fault Protection @5kHz/Fault checking/If Action Subsystem/Phase_B_Fault/Fault Check (Input OVP)_Phase_B ==
  note: "Von_Threshold" is set inside this state machine
  note: Fault Check (Input UVP)
  function : TriggerPort  TriggerType=function-call  VariantControl=(inherit)
  Chart1 : Stateflow chart  TreatAsAtomicUnit=on
  Data Store Read3 : DataStoreRead  DataStoreName=Vin_rms_Phase_B  IndexOptions=Index vector (dialog)  Indices=1  OutputSizes=1
  Data Store Write : DataStoreWrite  DataStoreName=Vin_OVP_Flag_Phase_B  IndexOptions=Index vector (dialog)  Indices=1  OutputSizes=1
  wires:
  Data Store Read3/1 -> Chart1/1(input)
  Chart1/1(Input_OVP_Flag) -> Data Store Write/1

== system CLA_Sample/Calibration,RMS, Fault Protection @5kHz/Fault checking/If Action Subsystem/Phase_B_Fault/Fault Check (Input UVP)_Phase_B ==
  note: "Von_Threshold" is set inside this state machine
  note: Fault Check (Input UVP)
  function : TriggerPort  TriggerType=function-call  VariantControl=(inherit)
  Chart1 : Stateflow chart  TreatAsAtomicUnit=on
  Data Store Read3 : DataStoreRead  DataStoreName=Vin_rms_Phase_B  IndexOptions=Index vector (dialog)  Indices=1  OutputSizes=1
  Data Store Write : DataStoreWrite  DataStoreName=Vin_UVP_Flag_Phase_B  IndexOptions=Index vector (dialog)  Indices=1  OutputSizes=1
  wires:
  Data Store Read3/1 -> Chart1/1(input)
  Chart1/1(Input_UVP_Flag) -> Data Store Write/1

== system CLA_Sample/Calibration,RMS, Fault Protection @5kHz/Fault checking/If Action Subsystem/Phase_B_Fault/Input current_OCP_Phase_B ==
  note: Output Voltage_Latch_OVP
  function : TriggerPort  TriggerType=function-call  VariantControl=(inherit)
  Abs : Abs  SaturateOnIntegerOverflow=off
  Chart2 : Stateflow chart  TreatAsAtomicUnit=on
  Data Store Read : DataStoreRead  DataStoreName=Inductor_Current_ADC_Phase_B  IndexOptions=Index vector (dialog)  Indices=1  OutputSizes=1
  Data Store Read1 : DataStoreRead  DataStoreName=Iin_OCP_Threshold  IndexOptions=Index vector (dialog)  Indices=1  OutputSizes=1
  Data Store Read3 : DataStoreRead  DataStoreName=Inductor_Current_1_65_ADC_Phase_B  IndexOptions=Index vector (dialog)  Indices=1  OutputSizes=1
  Data Store Write1 : DataStoreWrite  DataStoreName=Iin_OCP_Flag_phase_B  IndexOptions=Index vector (dialog)  Indices=1  OutputSizes=1
  Gain2 : Gain  Gain=0.00080586
  Gain3 : Gain  Gain=33.445
  Subtract2 : Sum  Inputs=+-
  wires:
  Data Store Read3/1 -> Subtract2/2
  Subtract2/1 -> Gain2/1
  Data Store Read/1 -> Subtract2/1
  Abs/1 -> Chart2/1(input_Iin)
  Chart2/1(Iin_OCP_Flag) -> Data Store Write1/1
  Data Store Read1/1 -> Chart2/2("OCP_Threshold ")
  Gain2/1 -> Gain3/1
  Gain3/1 -> Abs/1

== system CLA_Sample/Calibration,RMS, Fault Protection @5kHz/Fault checking/If Action Subsystem/Phase_C_Fault/Fault Check (Input OVP)_Phase_C ==
  note: "Von_Threshold" is set inside this state machine
  note: Fault Check (Input UVP)
  function : TriggerPort  TriggerType=function-call  VariantControl=(inherit)
  Chart1 : Stateflow chart  TreatAsAtomicUnit=on
  Data Store Read3 : DataStoreRead  DataStoreName=Vin_rms_Phase_C  IndexOptions=Index vector (dialog)  Indices=1  OutputSizes=1
  Data Store Write : DataStoreWrite  DataStoreName=Vin_OVP_Flag_Phase_C  IndexOptions=Index vector (dialog)  Indices=1  OutputSizes=1
  wires:
  Data Store Read3/1 -> Chart1/1(input)
  Chart1/1(Input_OVP_Flag) -> Data Store Write/1

== system CLA_Sample/Calibration,RMS, Fault Protection @5kHz/Fault checking/If Action Subsystem/Phase_C_Fault/Fault Check (Input UVP)_Phase_C ==
  note: "Von_Threshold" is set inside this state machine
  note: Fault Check (Input UVP)
  function : TriggerPort  TriggerType=function-call  VariantControl=(inherit)
  Chart1 : Stateflow chart  TreatAsAtomicUnit=on
  Data Store Read3 : DataStoreRead  DataStoreName=Vin_rms_Phase_C  IndexOptions=Index vector (dialog)  Indices=1  OutputSizes=1
  Data Store Write : DataStoreWrite  DataStoreName=Vin_UVP_Flag_Phase_C  IndexOptions=Index vector (dialog)  Indices=1  OutputSizes=1
  wires:
  Data Store Read3/1 -> Chart1/1(input)
  Chart1/1(Input_UVP_Flag) -> Data Store Write/1

== system CLA_Sample/Calibration,RMS, Fault Protection @5kHz/Fault checking/If Action Subsystem/Phase_C_Fault/Input current_OCP_Phase_C ==
  note: Output Voltage_Latch_OVP
  note: Vbulk_OVP_Threshold initialized in Data Store Memory
  function : TriggerPort  TriggerType=function-call  VariantControl=(inherit)
  Abs : Abs  SaturateOnIntegerOverflow=off
  Chart2 : Stateflow chart  TreatAsAtomicUnit=on
  Data Store Read : DataStoreRead  DataStoreName=Inductor_Current_ADC_Phase_C  IndexOptions=Index vector (dialog)  Indices=1  OutputSizes=1
  Data Store Read1 : DataStoreRead  DataStoreName=Iin_OCP_Threshold  IndexOptions=Index vector (dialog)  Indices=1  OutputSizes=1
  Data Store Read3 : DataStoreRead  DataStoreName=Inductor_Current_1_65_ADC_Phase_C  IndexOptions=Index vector (dialog)  Indices=1  OutputSizes=1
  Data Store Write1 : DataStoreWrite  DataStoreName=Iin_OCP_Flag_phase_C  IndexOptions=Index vector (dialog)  Indices=1  OutputSizes=1
  Gain2 : Gain  Gain=0.00080586
  Gain3 : Gain  Gain=33.445
  Subtract2 : Sum  Inputs=+-
  wires:
  Data Store Read3/1 -> Subtract2/2
  Subtract2/1 -> Gain2/1
  Data Store Read/1 -> Subtract2/1
  Abs/1 -> Chart2/1(input_Iin)
  Chart2/1(Iin_OCP_Flag) -> Data Store Write1/1
  Data Store Read1/1 -> Chart2/2("OCP_Threshold ")
  Gain2/1 -> Gain3/1
  Gain3/1 -> Abs/1

== system CLA_Sample/PWM Update @65KHz/Fixed Duty update_Phase_A/Archive/If Action Subsystem3/If Action Subsystem4 ==
  Action Port : ActionPort
  Data Store Read : DataStoreRead  DataStoreName=PWM_Duty_UART  IndexOptions=Index vector (dialog)  Indices=1  OutputSizes=1
  Data Store Read2 : DataStoreRead  DataStoreName=PWM_Duty_UART  IndexOptions=Index vector (dialog)  Indices=1  OutputSizes=1
  Data Store Read3 : DataStoreRead  DataStoreName=PFC_en_Phase_A  IndexOptions=Index vector (dialog)  Indices=1  OutputSizes=1
  Data Store Read4 : DataStoreRead  DataStoreName=One_Shot_Bar  IndexOptions=Index vector (dialog)  Indices=1  OutputSizes=1
  Data Store Write : DataStoreWrite  DataStoreName=PWM_DutyNearzero  IndexOptions=Index vector (dialog)  Indices=1  OutputSizes=1
  Product1 : Product  Inputs=3  OutDataTypeStr=double
  wires:
  Product1/1 -> Data Store Write/1
  Data Store Read3/1 -> Product1/1
  Data Store Read4/1 -> Product1/2
  Data Store Read2/1 -> Product1/3

== system CLA_Sample/PWM Update @65KHz/Fixed Duty update_Phase_A/Archive/If Action Subsystem3/If Action Subsystem5 ==
  Action Port : ActionPort
  Constant : Constant  Value=100
  Data Store Read : DataStoreRead  DataStoreName=PWM_Duty_UART  IndexOptions=Index vector (dialog)  Indices=1  OutputSizes=1
  Data Store Read2 : DataStoreRead  DataStoreName=PWM_Duty_UART  IndexOptions=Index vector (dialog)  Indices=1  OutputSizes=1
  Data Store Read3 : DataStoreRead  DataStoreName=PFC_en_Phase_A  IndexOptions=Index vector (dialog)  Indices=1  OutputSizes=1
  Data Store Read4 : DataStoreRead  DataStoreName=One_Shot_Bar  IndexOptions=Index vector (dialog)  Indices=1  OutputSizes=1
  Data Store Write : DataStoreWrite  DataStoreName=PWM_DutyNearzero  IndexOptions=Index vector (dialog)  Indices=1  OutputSizes=1
  Product1 : Product  Inputs=3  OutDataTypeStr=double
  Subtract : Sum  Inputs=+-
  wires:
  Data Store Read4/1 -> Product1/2
  Data Store Read3/1 -> Product1/1
  Data Store Read2/1 -> Product1/3
  Constant/1 -> Subtract/1
  Data Store Read/1 -> Subtract/2
  Product1/1 -> Data Store Write/1

== system CLA_Sample/PWM Update @65KHz/Fixed Duty update_Phase_B/Archive/If Action Subsystem3/If Action Subsystem4 ==
  Action Port : ActionPort
  Data Store Read : DataStoreRead  DataStoreName=PWM_Duty_UART  IndexOptions=Index vector (dialog)  Indices=1  OutputSizes=1
  Data Store Read2 : DataStoreRead  DataStoreName=PWM_Duty_UART  IndexOptions=Index vector (dialog)  Indices=1  OutputSizes=1
  Data Store Read3 : DataStoreRead  DataStoreName=PFC_en_Phase_A  IndexOptions=Index vector (dialog)  Indices=1  OutputSizes=1
  Data Store Read4 : DataStoreRead  DataStoreName=One_Shot_Bar  IndexOptions=Index vector (dialog)  Indices=1  OutputSizes=1
  Data Store Write : DataStoreWrite  DataStoreName=PWM_DutyNearzero  IndexOptions=Index vector (dialog)  Indices=1  OutputSizes=1
  Product1 : Product  Inputs=3  OutDataTypeStr=double
  wires:
  Product1/1 -> Data Store Write/1
  Data Store Read3/1 -> Product1/1
  Data Store Read4/1 -> Product1/2
  Data Store Read2/1 -> Product1/3
